simulink model "bpsk_simulink"  (R2024b)
settings: Solver=VariableStepAuto  StartTime=0.0  StopTime=10.0  RelTol=1e-3
libraries: commchan3 x1, commdigbbndpm3 x1, commsink2 x1, commrandsrc3 x1
settings Model: Creator=Ian  LastModifiedBy=Ian

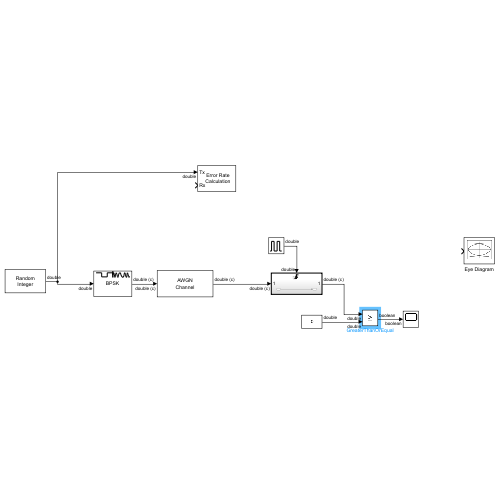
[thumbnail: Simulink's stored preview of the top-level diagram]
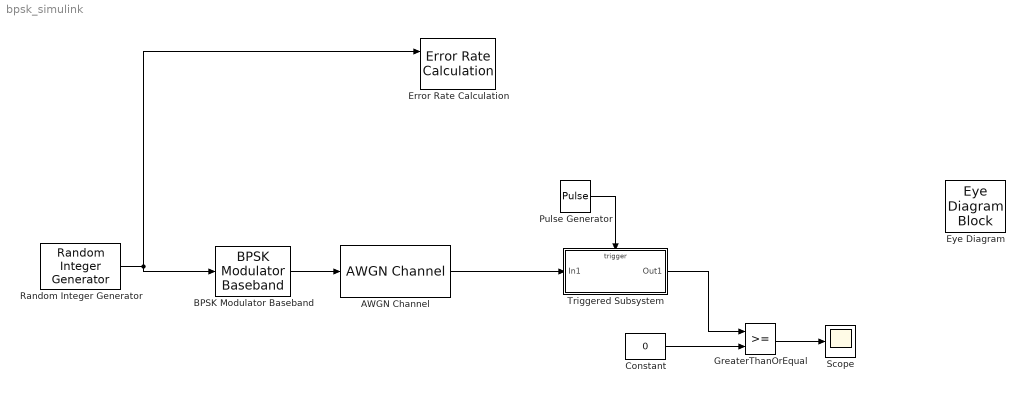
== system bpsk_simulink ==
  AWGN Channel : commchan3/AWGN Channel  LegacyMode=off  NoiseMethod="Signal to noise ratio  (SNR)"  noiseMode="Signal to noise ratio  (SNR)"  EbNo=10  EsNo=10  SNR=10  BitsPerSymbol=1  SignalPower=1  SamplesPerSymbol=1  SymbolPeriod=1  VarianceSource=Parameter  Variance=1  RandomStream=Global stream  Seed=67  SimulateUsing=Code generation
  BPSK Modulator Baseband : commdigbbndpm3/BPSK Modulator Baseband  Ph=0  outDtype=double  outWordLen=16  outUDDataType=sfix(16)  outFracLenMode=Best precision  outFracLen=15  outDataTypeStr=double  outLastDataTypeStr=double
  Constant : Constant  Value=0
  Error Rate Calculation : commsink2/Error Rate Calculation  N=0  st_delay=0  cp_mode=Entire frame  subframe=[]  PMode=Workspace  WsName=ErrorVec  RsMode2=off  stop=off  numErr=100  maxBits=1e6
  Eye Diagram : EyeDiagramBlock  WindowPosition=[880.000000,470.000000,800.000000,500.000000,]  ScopeFrameLocation=window
  GreaterThanOrEqual : RelationalOperator  OutDataTypeStr=boolean  RndMeth=Simplest  InputSameDT=off
  Pulse Generator : DiscretePulseGenerator  PulseType=Time based  Period=0.1  PulseWidth=50%
  Random Integer Generator : commrandsrc3/Random Integer Generator  SetSize=2  SeedSource=Auto  Seed=0  SampleTime=1  SamplesPerFrame=1  OutputDataType=double  SimulateUsing=Interpreted execution
  Scope : Scope
  Triggered Subsystem : Subsystem  TreatAsAtomicUnit=on
  wires:
  Constant/1 -> GreaterThanOrEqual/2
  Pulse Generator/1 -> Triggered Subsystem/Trigger
  Triggered Subsystem/1(Out1) -> GreaterThanOrEqual/1
  Random Integer Generator/1 -> Error Rate Calculation/1, BPSK Modulator Baseband/1
  BPSK Modulator Baseband/1 -> AWGN Channel/1
  AWGN Channel/1 -> Triggered Subsystem/1(In1)
  GreaterThanOrEqual/1 -> Scope/1

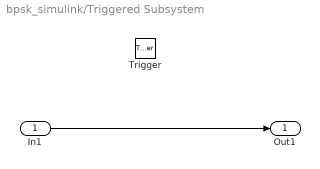
== system bpsk_simulink/Triggered Subsystem ==
  In1 : Inport
  Trigger : TriggerPort  VariantControl=(inherit)
  Out1 : Outport
  wires:
  In1/1 -> Out1/1
